simulink model "ieee80211n"  (Simulink 6.0)
settings: Solver=VariableStepDiscrete  StartTime=0.0  StopTime=inf  RelTol=1e-3
PreLoadFcn:
  | load IEEE80211n_init;
values from neighbouring files (symbols this model uses):
  params =     [IEEE80211n_init.mat]    (also in IEEE80211n_settings.m = p)
undefined symbols (not defined in the file or in its folder): magnitude
libraries: commblkintrlv2 x196, dspsigops x143, simulink x136, commdigbbndam2 x98, dspmtrx3 x96, dspsigattribs x69, dspstat3 x38, commutil2 x32, commsequence2 x26, commcnvcod2 x10, dspindex x9, dspmlti3 x8
(part 6 of 12)

== system ieee80211n/training sequence4/training sequence1 ==
  Frame Status Conversion1 : dspsigattribs/Frame Status Conversion  growRefPort=off  outframe=Frame-based
  Short Train sequence : Constant  Value=repmat(params.short_training_seq, [1 params.OFDM_LSTF_SymPerFrame])
  out : Outport
  wires:
  Short Train sequence/1 -> Frame Status Conversion1/1
  Frame Status Conversion1/1 -> out/1

== system ieee80211n/training sequence4/training sequence2 ==
  Frame Status Conversion{,1..3} (4 alike) : dspsigattribs/Frame Status Conversion  growRefPort=off  outframe=Frame-based
  "HT-LTF, 20MHz SS1" : Constant  Value=params.HT20_long_training_seq_ss1
  "HT-LTF, 20MHz SS2" : Constant  Value=params.HT20_long_training_seq_ss2
  "HT-LTF, 20MHz SS3" : Constant  Value=params.HT20_long_training_seq_ss3
  "HT-LTF, 20MHz SS4" : Constant  Value=params.HT20_long_training_seq_ss4
  "out, SS1" : Outport
  "out, SS2" : Outport  Port=2
  "out, SS3" : Outport  Port=3
  "out, SS4" : Outport  Port=4
  wires:
  "HT-LTF, 20MHz SS1"/1 -> Frame Status Conversion/1
  Frame Status Conversion/1 -> "out, SS1"/1
  "HT-LTF, 20MHz SS2"/1 -> Frame Status Conversion1/1
  Frame Status Conversion1/1 -> "out, SS2"/1
  "HT-LTF, 20MHz SS3"/1 -> Frame Status Conversion2/1
  Frame Status Conversion2/1 -> "out, SS3"/1
  "HT-LTF, 20MHz SS4"/1 -> Frame Status Conversion3/1
  Frame Status Conversion3/1 -> "out, SS4"/1

== system ieee80211n/training sequence4/training sequence3 ==
  Frame Status Conversion{,1..3} (4 alike) : dspsigattribs/Frame Status Conversion  growRefPort=off  outframe=Frame-based
  "HT-STF, 20MHz SS1" : Constant  Value=repmat(params.HT20_short_training_seq_ss1, [1 params.OFDM_HTSTF_SymPerFrame])
  "HT-STF, 20MHz SS2" : Constant  Value=repmat(params.HT20_short_training_seq_ss2, [1 params.OFDM_HTSTF_SymPerFrame])
  "HT-STF, 20MHz SS3" : Constant  Value=repmat(params.HT20_short_training_seq_ss3, [1 params.OFDM_HTSTF_SymPerFrame])
  "HT-STF, 20MHz SS4" : Constant  Value=repmat(params.HT20_short_training_seq_ss4, [1 params.OFDM_HTSTF_SymPerFrame])
  "out, SS1" : Outport
  "out, SS2" : Outport  Port=2
  "out, SS3" : Outport  Port=3
  "out, SS4" : Outport  Port=4
  wires:
  "HT-STF, 20MHz SS1"/1 -> Frame Status Conversion/1
  Frame Status Conversion/1 -> "out, SS1"/1
  "HT-STF, 20MHz SS2"/1 -> Frame Status Conversion1/1
  Frame Status Conversion1/1 -> "out, SS2"/1
  "HT-STF, 20MHz SS3"/1 -> Frame Status Conversion2/1
  Frame Status Conversion2/1 -> "out, SS3"/1
  "HT-STF, 20MHz SS4"/1 -> Frame Status Conversion3/1
  Frame Status Conversion3/1 -> "out, SS4"/1

== system ieee80211n/Demodbank/DecodeBankViterbi/Demodulator 1 ==
  rxsig : Inport  Port=1  LatchInput=off
  Enable : EnablePort
  Input bits : S-Function  AncestorBlock=dspindex/Multiport Selector  FunctionName=sdspmultiportsel  Parameters=rowsOrCols, numOutports, flatIdxVect, flatLenVect, idxErrMode  mask(Multiport Selector){rowsOrCols=Rows, idxCellArray={1:4*params.maxTxBitsPerBlock}, idxErrMode=Clip Index}
      mask prompts: rowsOrCols "Select:"; idxCellArray "Indices to output:"; idxErrMode "Invalid index:"
      mask help: Output specified rows or columns to one or more output ports. The number of output ports is determined by the number of index vectors, each specified as a separate vector entry in a cell array. Indices are 1-based and need not be unique.
      mask init:
      | [numOutports, flatLenVect, flatIdxVect] = dspblkmultiportsel(idxCellArray);
      mask Help: web(dspbhelp);
      mask StyleString: popup(Rows|Columns),edit,popup(Clip Index|Clip and Warn|Generate Error)
      mask Display: disp(['Select\n' &1]);
  Insert Zero1 : commsequence2/Insert Zero  insertZeroVector=punctureVector
  Insert Zero2 : commsequence2/Insert Zero  insertZeroVector=punctureVector
  Metric scaling : S-Function  AncestorBlock=dspindex/Multiport Selector  FunctionName=sdspmultiportsel  Parameters=rowsOrCols, numOutports, flatIdxVect, flatLenVect, idxErrMode  mask(Multiport Selector){rowsOrCols=Rows, idxCellArray={(1+4*params.maxTxBitsPerBlock):(2*4*params.maxTxBitsPerBlock)}, idxErrMode=Clip Index}
      mask prompts: rowsOrCols "Select:"; idxCellArray "Indices to output:"; idxErrMode "Invalid index:"
      mask help: Output specified rows or columns to one or more output ports. The number of output ports is determined by the number of index vectors, each specified as a separate vector entry in a cell array. Indices are 1-based and need not be unique.
      mask init:
      | [numOutports, flatLenVect, flatIdxVect] = dspblkmultiportsel(idxCellArray);
      mask Help: web(dspbhelp);
      mask StyleString: popup(Rows|Columns),edit,popup(Clip Index|Clip and Warn|Generate Error)
      mask Display: disp(['Select\n' &1]);
  Viterbi Decoder1 : S-Function  AncestorBlock=commcnvcod2/Viterbi Decoder  FunctionName=scomviterbi2  Parameters=S.k,S.n,S.numStates,S.outputs,S.nextStates, dectype, nsdecb, tbdepth, opmode, reset, mscale  mask(Viterbi Decoder){trellis=trellisStructure, dectype=Unquantized, nsdecb=4, tbdepth=vtbd, opmode=Continuous, reset=off, mscale=on}
      mask prompts: trellis "Trellis structure:"; dectype "Decision type:"; nsdecb "Number of soft decision bits:"; tbdepth "Traceback depth:"; opmode "Operation mode:"; reset "Reset input"; mscale "Use metric scaling input:"
      mask help: Uses the Viterbi algorithm to decode convolutionally encoded input data. Use the poly2trellis function to create a trellis using the constraint length, code generator (octal) and feedback connection (octal).
      mask init:
      | S= commblkviterbi(gcb,1,'init',trellis);
      | if ~isempty(S.status), error(S.status); end;
      | if opmode~=1, reset=0; end;
      mask Help: helpview(commbhelp)
      mask StyleString: edit,popup(Unquantized|Hard Decision|Soft Decision),edit,edit,popup(Continuous|Truncated|Terminated),checkbox,checkbox
      mask CallbackString: |commblkviterbi(gcb,1,'cbDecType');|||commblkviterbi(gcb,1,'cbOpMode');||
      mask Display:
      | plot(-5,-5,100,100,S.draw.x,S.draw.y);
      | disp('\nViterbi Decoder');
      | port_label('input',S.draw.p.i1,S.draw.p.i1s);
      | port_label('input',S.draw.p.i2,S.draw.p.i2s);
      | port_label('output',S.draw.p.o1,S.draw.p.o1s);
  Zero Pad2 : dspsigops/Zero Pad  padSigAt=End  zpadAlong=Columns  padNumOutRowsSpecMethod=User-specified  numOutRows=Nb  padNumOutColsSpecMethod=User-specified  numOutCols=1  trunc_flag=None
      settings: AttributesFormatString=\n
  Zero Pad3 : dspsigops/Zero Pad  padSigAt=End  zpadAlong=Columns  padNumOutRowsSpecMethod=User-specified  numOutRows=Nb  padNumOutColsSpecMethod=User-specified  numOutCols=1  trunc_flag=None
      settings: AttributesFormatString=\n
  rxdata : Outport  OutputWhenDisabled=reset  InitialOutput=0
  wires:
  Viterbi Decoder1/1 -> rxdata/1
  Zero Pad2/1 -> Insert Zero1/1
  Input bits/1 -> Zero Pad2/1
  Zero Pad3/1 -> Insert Zero2/1
  Metric scaling/1 -> Zero Pad3/1
  Insert Zero1/1 -> Viterbi Decoder1/1
  rxsig/1 -> Input bits/1, Metric scaling/1
  Insert Zero2/1 -> Viterbi Decoder1/2

== system ieee80211n/Demodbank/DecodeBankViterbi/Demodulator 2 ==
  rxsig : Inport  Port=1  LatchInput=off
  Enable : EnablePort
  Input bits : S-Function  AncestorBlock=dspindex/Multiport Selector  FunctionName=sdspmultiportsel  Parameters=rowsOrCols, numOutports, flatIdxVect, flatLenVect, idxErrMode  mask(Multiport Selector){rowsOrCols=Rows, idxCellArray={1:4*params.maxTxBitsPerBlock}, idxErrMode=Clip Index}
      mask prompts: rowsOrCols "Select:"; idxCellArray "Indices to output:"; idxErrMode "Invalid index:"
      mask help: Output specified rows or columns to one or more output ports. The number of output ports is determined by the number of index vectors, each specified as a separate vector entry in a cell array. Indices are 1-based and need not be unique.
      mask init:
      | [numOutports, flatLenVect, flatIdxVect] = dspblkmultiportsel(idxCellArray);
      mask Help: web(dspbhelp);
      mask StyleString: popup(Rows|Columns),edit,popup(Clip Index|Clip and Warn|Generate Error)
      mask Display: disp(['Select\n' &1]);
  Insert Zero1 : commsequence2/Insert Zero  insertZeroVector=punctureVector
  Insert Zero2 : commsequence2/Insert Zero  insertZeroVector=punctureVector
  Metric scaling : S-Function  AncestorBlock=dspindex/Multiport Selector  FunctionName=sdspmultiportsel  Parameters=rowsOrCols, numOutports, flatIdxVect, flatLenVect, idxErrMode  mask(Multiport Selector){rowsOrCols=Rows, idxCellArray={(1+4*params.maxTxBitsPerBlock):(2*4*params.maxTxBitsPerBlock)}, idxErrMode=Clip Index}
      mask prompts: rowsOrCols "Select:"; idxCellArray "Indices to output:"; idxErrMode "Invalid index:"
      mask help: Output specified rows or columns to one or more output ports. The number of output ports is determined by the number of index vectors, each specified as a separate vector entry in a cell array. Indices are 1-based and need not be unique.
      mask init:
      | [numOutports, flatLenVect, flatIdxVect] = dspblkmultiportsel(idxCellArray);
      mask Help: web(dspbhelp);
      mask StyleString: popup(Rows|Columns),edit,popup(Clip Index|Clip and Warn|Generate Error)
      mask Display: disp(['Select\n' &1]);
  Viterbi Decoder1 : S-Function  AncestorBlock=commcnvcod2/Viterbi Decoder  FunctionName=scomviterbi2  Parameters=S.k,S.n,S.numStates,S.outputs,S.nextStates, dectype, nsdecb, tbdepth, opmode, reset, mscale  mask(Viterbi Decoder){trellis=trellisStructure, dectype=Unquantized, nsdecb=4, tbdepth=vtbd, opmode=Continuous, reset=off, mscale=on}
      mask prompts: trellis "Trellis structure:"; dectype "Decision type:"; nsdecb "Number of soft decision bits:"; tbdepth "Traceback depth:"; opmode "Operation mode:"; reset "Reset input"; mscale "Use metric scaling input:"
      mask help: Uses the Viterbi algorithm to decode convolutionally encoded input data. Use the poly2trellis function to create a trellis using the constraint length, code generator (octal) and feedback connection (octal).
      mask init:
      | S= commblkviterbi(gcb,1,'init',trellis);
      | if ~isempty(S.status), error(S.status); end;
      | if opmode~=1, reset=0; end;
      mask Help: helpview(commbhelp)
      mask StyleString: edit,popup(Unquantized|Hard Decision|Soft Decision),edit,edit,popup(Continuous|Truncated|Terminated),checkbox,checkbox
      mask CallbackString: |commblkviterbi(gcb,1,'cbDecType');|||commblkviterbi(gcb,1,'cbOpMode');||
      mask Display:
      | plot(-5,-5,100,100,S.draw.x,S.draw.y);
      | disp('\nViterbi Decoder');
      | port_label('input',S.draw.p.i1,S.draw.p.i1s);
      | port_label('input',S.draw.p.i2,S.draw.p.i2s);
      | port_label('output',S.draw.p.o1,S.draw.p.o1s);
  Zero Pad2 : dspsigops/Zero Pad  padSigAt=End  zpadAlong=Columns  padNumOutRowsSpecMethod=User-specified  numOutRows=Nb  padNumOutColsSpecMethod=User-specified  numOutCols=1  trunc_flag=None
      settings: AttributesFormatString=\n
  Zero Pad3 : dspsigops/Zero Pad  padSigAt=End  zpadAlong=Columns  padNumOutRowsSpecMethod=User-specified  numOutRows=Nb  padNumOutColsSpecMethod=User-specified  numOutCols=1  trunc_flag=None
      settings: AttributesFormatString=\n
  rxdata : Outport  OutputWhenDisabled=reset  InitialOutput=0
  wires:
  Viterbi Decoder1/1 -> rxdata/1
  Zero Pad2/1 -> Insert Zero1/1
  Input bits/1 -> Zero Pad2/1
  Zero Pad3/1 -> Insert Zero2/1
  Metric scaling/1 -> Zero Pad3/1
  Insert Zero1/1 -> Viterbi Decoder1/1
  rxsig/1 -> Input bits/1, Metric scaling/1
  Insert Zero2/1 -> Viterbi Decoder1/2

== system ieee80211n/Demodbank/DecodeBankViterbi/Demodulator 3 ==
  rxsig : Inport  Port=1  LatchInput=off
  Enable : EnablePort
  Input bits : S-Function  AncestorBlock=dspindex/Multiport Selector  FunctionName=sdspmultiportsel  Parameters=rowsOrCols, numOutports, flatIdxVect, flatLenVect, idxErrMode  mask(Multiport Selector){rowsOrCols=Rows, idxCellArray={1:4*params.maxTxBitsPerBlock}, idxErrMode=Clip Index}
      mask prompts: rowsOrCols "Select:"; idxCellArray "Indices to output:"; idxErrMode "Invalid index:"
      mask help: Output specified rows or columns to one or more output ports. The number of output ports is determined by the number of index vectors, each specified as a separate vector entry in a cell array. Indices are 1-based and need not be unique.
      mask init:
      | [numOutports, flatLenVect, flatIdxVect] = dspblkmultiportsel(idxCellArray);
      mask Help: web(dspbhelp);
      mask StyleString: popup(Rows|Columns),edit,popup(Clip Index|Clip and Warn|Generate Error)
      mask Display: disp(['Select\n' &1]);
  Insert Zero1 : commsequence2/Insert Zero  insertZeroVector=punctureVector
  Insert Zero2 : commsequence2/Insert Zero  insertZeroVector=punctureVector
  Metric scaling : S-Function  AncestorBlock=dspindex/Multiport Selector  FunctionName=sdspmultiportsel  Parameters=rowsOrCols, numOutports, flatIdxVect, flatLenVect, idxErrMode  mask(Multiport Selector){rowsOrCols=Rows, idxCellArray={(1+4*params.maxTxBitsPerBlock):(2*4*params.maxTxBitsPerBlock)}, idxErrMode=Clip Index}
      mask prompts: rowsOrCols "Select:"; idxCellArray "Indices to output:"; idxErrMode "Invalid index:"
      mask help: Output specified rows or columns to one or more output ports. The number of output ports is determined by the number of index vectors, each specified as a separate vector entry in a cell array. Indices are 1-based and need not be unique.
      mask init:
      | [numOutports, flatLenVect, flatIdxVect] = dspblkmultiportsel(idxCellArray);
      mask Help: web(dspbhelp);
      mask StyleString: popup(Rows|Columns),edit,popup(Clip Index|Clip and Warn|Generate Error)
      mask Display: disp(['Select\n' &1]);
  Viterbi Decoder1 : S-Function  AncestorBlock=commcnvcod2/Viterbi Decoder  FunctionName=scomviterbi2  Parameters=S.k,S.n,S.numStates,S.outputs,S.nextStates, dectype, nsdecb, tbdepth, opmode, reset, mscale  mask(Viterbi Decoder){trellis=trellisStructure, dectype=Unquantized, nsdecb=4, tbdepth=vtbd, opmode=Continuous, reset=off, mscale=on}
      mask prompts: trellis "Trellis structure:"; dectype "Decision type:"; nsdecb "Number of soft decision bits:"; tbdepth "Traceback depth:"; opmode "Operation mode:"; reset "Reset input"; mscale "Use metric scaling input:"
      mask help: Uses the Viterbi algorithm to decode convolutionally encoded input data. Use the poly2trellis function to create a trellis using the constraint length, code generator (octal) and feedback connection (octal).
      mask init:
      | S= commblkviterbi(gcb,1,'init',trellis);
      | if ~isempty(S.status), error(S.status); end;
      | if opmode~=1, reset=0; end;
      mask Help: helpview(commbhelp)
      mask StyleString: edit,popup(Unquantized|Hard Decision|Soft Decision),edit,edit,popup(Continuous|Truncated|Terminated),checkbox,checkbox
      mask CallbackString: |commblkviterbi(gcb,1,'cbDecType');|||commblkviterbi(gcb,1,'cbOpMode');||
      mask Display:
      | plot(-5,-5,100,100,S.draw.x,S.draw.y);
      | disp('\nViterbi Decoder');
      | port_label('input',S.draw.p.i1,S.draw.p.i1s);
      | port_label('input',S.draw.p.i2,S.draw.p.i2s);
      | port_label('output',S.draw.p.o1,S.draw.p.o1s);
  Zero Pad2 : dspsigops/Zero Pad  padSigAt=End  zpadAlong=Columns  padNumOutRowsSpecMethod=User-specified  numOutRows=Nb  padNumOutColsSpecMethod=User-specified  numOutCols=1  trunc_flag=None
      settings: AttributesFormatString=\n
  Zero Pad3 : dspsigops/Zero Pad  padSigAt=End  zpadAlong=Columns  padNumOutRowsSpecMethod=User-specified  numOutRows=Nb  padNumOutColsSpecMethod=User-specified  numOutCols=1  trunc_flag=None
      settings: AttributesFormatString=\n
  rxdata : Outport  OutputWhenDisabled=reset  InitialOutput=0
  wires:
  Viterbi Decoder1/1 -> rxdata/1
  Zero Pad2/1 -> Insert Zero1/1
  Input bits/1 -> Zero Pad2/1
  Zero Pad3/1 -> Insert Zero2/1
  Metric scaling/1 -> Zero Pad3/1
  Insert Zero1/1 -> Viterbi Decoder1/1
  rxsig/1 -> Input bits/1, Metric scaling/1
  Insert Zero2/1 -> Viterbi Decoder1/2

== system ieee80211n/Demodbank/DecodeBankViterbi/Demodulator 4 ==
  rxsig : Inport  Port=1  LatchInput=off
  Enable : EnablePort
  Input bits : S-Function  AncestorBlock=dspindex/Multiport Selector  FunctionName=sdspmultiportsel  Parameters=rowsOrCols, numOutports, flatIdxVect, flatLenVect, idxErrMode  mask(Multiport Selector){rowsOrCols=Rows, idxCellArray={1:4*params.maxTxBitsPerBlock}, idxErrMode=Clip Index}
      mask prompts: rowsOrCols "Select:"; idxCellArray "Indices to output:"; idxErrMode "Invalid index:"
      mask help: Output specified rows or columns to one or more output ports. The number of output ports is determined by the number of index vectors, each specified as a separate vector entry in a cell array. Indices are 1-based and need not be unique.
      mask init:
      | [numOutports, flatLenVect, flatIdxVect] = dspblkmultiportsel(idxCellArray);
      mask Help: web(dspbhelp);
      mask StyleString: popup(Rows|Columns),edit,popup(Clip Index|Clip and Warn|Generate Error)
      mask Display: disp(['Select\n' &1]);
  Insert Zero1 : commsequence2/Insert Zero  insertZeroVector=punctureVector
  Insert Zero2 : commsequence2/Insert Zero  insertZeroVector=punctureVector
  Metric scaling : S-Function  AncestorBlock=dspindex/Multiport Selector  FunctionName=sdspmultiportsel  Parameters=rowsOrCols, numOutports, flatIdxVect, flatLenVect, idxErrMode  mask(Multiport Selector){rowsOrCols=Rows, idxCellArray={(1+4*params.maxTxBitsPerBlock):(2*4*params.maxTxBitsPerBlock)}, idxErrMode=Clip Index}
      mask prompts: rowsOrCols "Select:"; idxCellArray "Indices to output:"; idxErrMode "Invalid index:"
      mask help: Output specified rows or columns to one or more output ports. The number of output ports is determined by the number of index vectors, each specified as a separate vector entry in a cell array. Indices are 1-based and need not be unique.
      mask init:
      | [numOutports, flatLenVect, flatIdxVect] = dspblkmultiportsel(idxCellArray);
      mask Help: web(dspbhelp);
      mask StyleString: popup(Rows|Columns),edit,popup(Clip Index|Clip and Warn|Generate Error)
      mask Display: disp(['Select\n' &1]);
  Viterbi Decoder1 : S-Function  AncestorBlock=commcnvcod2/Viterbi Decoder  FunctionName=scomviterbi2  Parameters=S.k,S.n,S.numStates,S.outputs,S.nextStates, dectype, nsdecb, tbdepth, opmode, reset, mscale  mask(Viterbi Decoder){trellis=trellisStructure, dectype=Unquantized, nsdecb=4, tbdepth=vtbd, opmode=Continuous, reset=off, mscale=on}
      mask prompts: trellis "Trellis structure:"; dectype "Decision type:"; nsdecb "Number of soft decision bits:"; tbdepth "Traceback depth:"; opmode "Operation mode:"; reset "Reset input"; mscale "Use metric scaling input:"
      mask help: Uses the Viterbi algorithm to decode convolutionally encoded input data. Use the poly2trellis function to create a trellis using the constraint length, code generator (octal) and feedback connection (octal).
      mask init:
      | S= commblkviterbi(gcb,1,'init',trellis);
      | if ~isempty(S.status), error(S.status); end;
      | if opmode~=1, reset=0; end;
      mask Help: helpview(commbhelp)
      mask StyleString: edit,popup(Unquantized|Hard Decision|Soft Decision),edit,edit,popup(Continuous|Truncated|Terminated),checkbox,checkbox
      mask CallbackString: |commblkviterbi(gcb,1,'cbDecType');|||commblkviterbi(gcb,1,'cbOpMode');||
      mask Display:
      | plot(-5,-5,100,100,S.draw.x,S.draw.y);
      | disp('\nViterbi Decoder');
      | port_label('input',S.draw.p.i1,S.draw.p.i1s);
      | port_label('input',S.draw.p.i2,S.draw.p.i2s);
      | port_label('output',S.draw.p.o1,S.draw.p.o1s);
  Zero Pad2 : dspsigops/Zero Pad  padSigAt=End  zpadAlong=Columns  padNumOutRowsSpecMethod=User-specified  numOutRows=Nb  padNumOutColsSpecMethod=User-specified  numOutCols=1  trunc_flag=None
      settings: AttributesFormatString=\n
  Zero Pad3 : dspsigops/Zero Pad  padSigAt=End  zpadAlong=Columns  padNumOutRowsSpecMethod=User-specified  numOutRows=Nb  padNumOutColsSpecMethod=User-specified  numOutCols=1  trunc_flag=None
      settings: AttributesFormatString=\n
  rxdata : Outport  OutputWhenDisabled=reset  InitialOutput=0
  wires:
  Viterbi Decoder1/1 -> rxdata/1
  rxsig/1 -> Input bits/1, Metric scaling/1
  Zero Pad2/1 -> Insert Zero1/1
  Input bits/1 -> Zero Pad2/1
  Zero Pad3/1 -> Insert Zero2/1
  Metric scaling/1 -> Zero Pad3/1
  Insert Zero1/1 -> Viterbi Decoder1/1
  Insert Zero2/1 -> Viterbi Decoder1/2

== system ieee80211n/Demodbank/DecodeBankViterbi/Demodulator 5 ==
  rxsig : Inport  Port=1  LatchInput=off
  Enable : EnablePort
  Input bits : S-Function  AncestorBlock=dspindex/Multiport Selector  FunctionName=sdspmultiportsel  Parameters=rowsOrCols, numOutports, flatIdxVect, flatLenVect, idxErrMode  mask(Multiport Selector){rowsOrCols=Rows, idxCellArray={1:4*params.maxTxBitsPerBlock}, idxErrMode=Clip Index}
      mask prompts: rowsOrCols "Select:"; idxCellArray "Indices to output:"; idxErrMode "Invalid index:"
      mask help: Output specified rows or columns to one or more output ports. The number of output ports is determined by the number of index vectors, each specified as a separate vector entry in a cell array. Indices are 1-based and need not be unique.
      mask init:
      | [numOutports, flatLenVect, flatIdxVect] = dspblkmultiportsel(idxCellArray);
      mask Help: web(dspbhelp);
      mask StyleString: popup(Rows|Columns),edit,popup(Clip Index|Clip and Warn|Generate Error)
      mask Display: disp(['Select\n' &1]);
  Insert Zero1 : commsequence2/Insert Zero  insertZeroVector=punctureVector
  Insert Zero2 : commsequence2/Insert Zero  insertZeroVector=punctureVector
  Metric scaling : S-Function  AncestorBlock=dspindex/Multiport Selector  FunctionName=sdspmultiportsel  Parameters=rowsOrCols, numOutports, flatIdxVect, flatLenVect, idxErrMode  mask(Multiport Selector){rowsOrCols=Rows, idxCellArray={(1+4*params.maxTxBitsPerBlock):(2*4*params.maxTxBitsPerBlock)}, idxErrMode=Clip Index}
      mask prompts: rowsOrCols "Select:"; idxCellArray "Indices to output:"; idxErrMode "Invalid index:"
      mask help: Output specified rows or columns to one or more output ports. The number of output ports is determined by the number of index vectors, each specified as a separate vector entry in a cell array. Indices are 1-based and need not be unique.
      mask init:
      | [numOutports, flatLenVect, flatIdxVect] = dspblkmultiportsel(idxCellArray);
      mask Help: web(dspbhelp);
      mask StyleString: popup(Rows|Columns),edit,popup(Clip Index|Clip and Warn|Generate Error)
      mask Display: disp(['Select\n' &1]);
  Viterbi Decoder1 : S-Function  AncestorBlock=commcnvcod2/Viterbi Decoder  FunctionName=scomviterbi2  Parameters=S.k,S.n,S.numStates,S.outputs,S.nextStates, dectype, nsdecb, tbdepth, opmode, reset, mscale  mask(Viterbi Decoder){trellis=trellisStructure, dectype=Unquantized, nsdecb=4, tbdepth=vtbd, opmode=Continuous, reset=off, mscale=on}
      mask prompts: trellis "Trellis structure:"; dectype "Decision type:"; nsdecb "Number of soft decision bits:"; tbdepth "Traceback depth:"; opmode "Operation mode:"; reset "Reset input"; mscale "Use metric scaling input:"
      mask help: Uses the Viterbi algorithm to decode convolutionally encoded input data. Use the poly2trellis function to create a trellis using the constraint length, code generator (octal) and feedback connection (octal).
      mask init:
      | S= commblkviterbi(gcb,1,'init',trellis);
      | if ~isempty(S.status), error(S.status); end;
      | if opmode~=1, reset=0; end;
      mask Help: helpview(commbhelp)
      mask StyleString: edit,popup(Unquantized|Hard Decision|Soft Decision),edit,edit,popup(Continuous|Truncated|Terminated),checkbox,checkbox
      mask CallbackString: |commblkviterbi(gcb,1,'cbDecType');|||commblkviterbi(gcb,1,'cbOpMode');||
      mask Display:
      | plot(-5,-5,100,100,S.draw.x,S.draw.y);
      | disp('\nViterbi Decoder');
      | port_label('input',S.draw.p.i1,S.draw.p.i1s);
      | port_label('input',S.draw.p.i2,S.draw.p.i2s);
      | port_label('output',S.draw.p.o1,S.draw.p.o1s);
  Zero Pad2 : dspsigops/Zero Pad  padSigAt=End  zpadAlong=Columns  padNumOutRowsSpecMethod=User-specified  numOutRows=Nb  padNumOutColsSpecMethod=User-specified  numOutCols=1  trunc_flag=None
      settings: AttributesFormatString=\n
  Zero Pad3 : dspsigops/Zero Pad  padSigAt=End  zpadAlong=Columns  padNumOutRowsSpecMethod=User-specified  numOutRows=Nb  padNumOutColsSpecMethod=User-specified  numOutCols=1  trunc_flag=None
      settings: AttributesFormatString=\n
  rxdata : Outport  OutputWhenDisabled=reset  InitialOutput=0
  wires:
  Viterbi Decoder1/1 -> rxdata/1
  rxsig/1 -> Input bits/1, Metric scaling/1
  Zero Pad2/1 -> Insert Zero1/1
  Input bits/1 -> Zero Pad2/1
  Zero Pad3/1 -> Insert Zero2/1
  Metric scaling/1 -> Zero Pad3/1
  Insert Zero1/1 -> Viterbi Decoder1/1
  Insert Zero2/1 -> Viterbi Decoder1/2

== system ieee80211n/Demodbank/DecodeBankViterbi/Demodulator 6 ==
  rxsig : Inport  Port=1  LatchInput=off
  Enable : EnablePort
  Input bits : S-Function  AncestorBlock=dspindex/Multiport Selector  FunctionName=sdspmultiportsel  Parameters=rowsOrCols, numOutports, flatIdxVect, flatLenVect, idxErrMode  mask(Multiport Selector){rowsOrCols=Rows, idxCellArray={1:4*params.maxTxBitsPerBlock}, idxErrMode=Clip Index}
      mask prompts: rowsOrCols "Select:"; idxCellArray "Indices to output:"; idxErrMode "Invalid index:"
      mask help: Output specified rows or columns to one or more output ports. The number of output ports is determined by the number of index vectors, each specified as a separate vector entry in a cell array. Indices are 1-based and need not be unique.
      mask init:
      | [numOutports, flatLenVect, flatIdxVect] = dspblkmultiportsel(idxCellArray);
      mask Help: web(dspbhelp);
      mask StyleString: popup(Rows|Columns),edit,popup(Clip Index|Clip and Warn|Generate Error)
      mask Display: disp(['Select\n' &1]);
  Insert Zero1 : commsequence2/Insert Zero  insertZeroVector=punctureVector
  Insert Zero2 : commsequence2/Insert Zero  insertZeroVector=punctureVector
  Metric scaling : S-Function  AncestorBlock=dspindex/Multiport Selector  FunctionName=sdspmultiportsel  Parameters=rowsOrCols, numOutports, flatIdxVect, flatLenVect, idxErrMode  mask(Multiport Selector){rowsOrCols=Rows, idxCellArray={(1+4*params.maxTxBitsPerBlock):(2*4*params.maxTxBitsPerBlock)}, idxErrMode=Clip Index}
      mask prompts: rowsOrCols "Select:"; idxCellArray "Indices to output:"; idxErrMode "Invalid index:"
      mask help: Output specified rows or columns to one or more output ports. The number of output ports is determined by the number of index vectors, each specified as a separate vector entry in a cell array. Indices are 1-based and need not be unique.
      mask init:
      | [numOutports, flatLenVect, flatIdxVect] = dspblkmultiportsel(idxCellArray);
      mask Help: web(dspbhelp);
      mask StyleString: popup(Rows|Columns),edit,popup(Clip Index|Clip and Warn|Generate Error)
      mask Display: disp(['Select\n' &1]);
  Viterbi Decoder1 : S-Function  AncestorBlock=commcnvcod2/Viterbi Decoder  FunctionName=scomviterbi2  Parameters=S.k,S.n,S.numStates,S.outputs,S.nextStates, dectype, nsdecb, tbdepth, opmode, reset, mscale  mask(Viterbi Decoder){trellis=trellisStructure, dectype=Unquantized, nsdecb=4, tbdepth=vtbd, opmode=Continuous, reset=off, mscale=on}
      mask prompts: trellis "Trellis structure:"; dectype "Decision type:"; nsdecb "Number of soft decision bits:"; tbdepth "Traceback depth:"; opmode "Operation mode:"; reset "Reset input"; mscale "Use metric scaling input:"
      mask help: Uses the Viterbi algorithm to decode convolutionally encoded input data. Use the poly2trellis function to create a trellis using the constraint length, code generator (octal) and feedback connection (octal).
      mask init:
      | S= commblkviterbi(gcb,1,'init',trellis);
      | if ~isempty(S.status), error(S.status); end;
      | if opmode~=1, reset=0; end;
      mask Help: helpview(commbhelp)
      mask StyleString: edit,popup(Unquantized|Hard Decision|Soft Decision),edit,edit,popup(Continuous|Truncated|Terminated),checkbox,checkbox
      mask CallbackString: |commblkviterbi(gcb,1,'cbDecType');|||commblkviterbi(gcb,1,'cbOpMode');||
      mask Display:
      | plot(-5,-5,100,100,S.draw.x,S.draw.y);
      | disp('\nViterbi Decoder');
      | port_label('input',S.draw.p.i1,S.draw.p.i1s);
      | port_label('input',S.draw.p.i2,S.draw.p.i2s);
      | port_label('output',S.draw.p.o1,S.draw.p.o1s);
  Zero Pad2 : dspsigops/Zero Pad  padSigAt=End  zpadAlong=Columns  padNumOutRowsSpecMethod=User-specified  numOutRows=Nb  padNumOutColsSpecMethod=User-specified  numOutCols=1  trunc_flag=None
      settings: AttributesFormatString=\n
  Zero Pad3 : dspsigops/Zero Pad  padSigAt=End  zpadAlong=Columns  padNumOutRowsSpecMethod=User-specified  numOutRows=Nb  padNumOutColsSpecMethod=User-specified  numOutCols=1  trunc_flag=None
      settings: AttributesFormatString=\n
  rxdata : Outport  OutputWhenDisabled=reset  InitialOutput=0
  wires:
  Viterbi Decoder1/1 -> rxdata/1
  Zero Pad2/1 -> Insert Zero1/1
  Input bits/1 -> Zero Pad2/1
  Zero Pad3/1 -> Insert Zero2/1
  Metric scaling/1 -> Zero Pad3/1
  Insert Zero1/1 -> Viterbi Decoder1/1
  rxsig/1 -> Input bits/1, Metric scaling/1
  Insert Zero2/1 -> Viterbi Decoder1/2

== system ieee80211n/Demodbank/DecodeBankViterbi/Demodulator 7 ==
  rxsig : Inport  Port=1  LatchInput=off
  Enable : EnablePort
  Input bits : S-Function  AncestorBlock=dspindex/Multiport Selector  FunctionName=sdspmultiportsel  Parameters=rowsOrCols, numOutports, flatIdxVect, flatLenVect, idxErrMode  mask(Multiport Selector){rowsOrCols=Rows, idxCellArray={1:4*params.maxTxBitsPerBlock}, idxErrMode=Clip Index}
      mask prompts: rowsOrCols "Select:"; idxCellArray "Indices to output:"; idxErrMode "Invalid index:"
      mask help: Output specified rows or columns to one or more output ports. The number of output ports is determined by the number of index vectors, each specified as a separate vector entry in a cell array. Indices are 1-based and need not be unique.
      mask init:
      | [numOutports, flatLenVect, flatIdxVect] = dspblkmultiportsel(idxCellArray);
      mask Help: web(dspbhelp);
      mask StyleString: popup(Rows|Columns),edit,popup(Clip Index|Clip and Warn|Generate Error)
      mask Display: disp(['Select\n' &1]);
  Insert Zero1 : commsequence2/Insert Zero  insertZeroVector=punctureVector
  Insert Zero2 : commsequence2/Insert Zero  insertZeroVector=punctureVector
  Metric scaling : S-Function  AncestorBlock=dspindex/Multiport Selector  FunctionName=sdspmultiportsel  Parameters=rowsOrCols, numOutports, flatIdxVect, flatLenVect, idxErrMode  mask(Multiport Selector){rowsOrCols=Rows, idxCellArray={(1+4*params.maxTxBitsPerBlock):(2*4*params.maxTxBitsPerBlock)}, idxErrMode=Clip Index}
      mask prompts: rowsOrCols "Select:"; idxCellArray "Indices to output:"; idxErrMode "Invalid index:"
      mask help: Output specified rows or columns to one or more output ports. The number of output ports is determined by the number of index vectors, each specified as a separate vector entry in a cell array. Indices are 1-based and need not be unique.
      mask init:
      | [numOutports, flatLenVect, flatIdxVect] = dspblkmultiportsel(idxCellArray);
      mask Help: web(dspbhelp);
      mask StyleString: popup(Rows|Columns),edit,popup(Clip Index|Clip and Warn|Generate Error)
      mask Display: disp(['Select\n' &1]);
  Viterbi Decoder1 : S-Function  AncestorBlock=commcnvcod2/Viterbi Decoder  FunctionName=scomviterbi2  Parameters=S.k,S.n,S.numStates,S.outputs,S.nextStates, dectype, nsdecb, tbdepth, opmode, reset, mscale  mask(Viterbi Decoder){trellis=trellisStructure, dectype=Unquantized, nsdecb=4, tbdepth=vtbd, opmode=Continuous, reset=off, mscale=on}
      mask prompts: trellis "Trellis structure:"; dectype "Decision type:"; nsdecb "Number of soft decision bits:"; tbdepth "Traceback depth:"; opmode "Operation mode:"; reset "Reset input"; mscale "Use metric scaling input:"
      mask help: Uses the Viterbi algorithm to decode convolutionally encoded input data. Use the poly2trellis function to create a trellis using the constraint length, code generator (octal) and feedback connection (octal).
      mask init:
      | S= commblkviterbi(gcb,1,'init',trellis);
      | if ~isempty(S.status), error(S.status); end;
      | if opmode~=1, reset=0; end;
      mask Help: helpview(commbhelp)
      mask StyleString: edit,popup(Unquantized|Hard Decision|Soft Decision),edit,edit,popup(Continuous|Truncated|Terminated),checkbox,checkbox
      mask CallbackString: |commblkviterbi(gcb,1,'cbDecType');|||commblkviterbi(gcb,1,'cbOpMode');||
      mask Display:
      | plot(-5,-5,100,100,S.draw.x,S.draw.y);
      | disp('\nViterbi Decoder');
      | port_label('input',S.draw.p.i1,S.draw.p.i1s);
      | port_label('input',S.draw.p.i2,S.draw.p.i2s);
      | port_label('output',S.draw.p.o1,S.draw.p.o1s);
  Zero Pad2 : dspsigops/Zero Pad  padSigAt=End  zpadAlong=Columns  padNumOutRowsSpecMethod=User-specified  numOutRows=Nb  padNumOutColsSpecMethod=User-specified  numOutCols=1  trunc_flag=None
      settings: AttributesFormatString=\n
  Zero Pad3 : dspsigops/Zero Pad  padSigAt=End  zpadAlong=Columns  padNumOutRowsSpecMethod=User-specified  numOutRows=Nb  padNumOutColsSpecMethod=User-specified  numOutCols=1  trunc_flag=None
      settings: AttributesFormatString=\n
  rxdata : Outport  OutputWhenDisabled=reset  InitialOutput=0
  wires:
  Viterbi Decoder1/1 -> rxdata/1
  Zero Pad2/1 -> Insert Zero1/1
  Input bits/1 -> Zero Pad2/1
  Zero Pad3/1 -> Insert Zero2/1
  Metric scaling/1 -> Zero Pad3/1
  Insert Zero1/1 -> Viterbi Decoder1/1
  rxsig/1 -> Input bits/1, Metric scaling/1
  Insert Zero2/1 -> Viterbi Decoder1/2

== system ieee80211n/Demodbank/DecodeBankViterbi/Demodulator 8 ==
  rxsig : Inport  Port=1  LatchInput=off
  Enable : EnablePort
  Input bits : S-Function  AncestorBlock=dspindex/Multiport Selector  FunctionName=sdspmultiportsel  Parameters=rowsOrCols, numOutports, flatIdxVect, flatLenVect, idxErrMode  mask(Multiport Selector){rowsOrCols=Rows, idxCellArray={1:4*params.maxTxBitsPerBlock}, idxErrMode=Clip Index}
      mask prompts: rowsOrCols "Select:"; idxCellArray "Indices to output:"; idxErrMode "Invalid index:"
      mask help: Output specified rows or columns to one or more output ports. The number of output ports is determined by the number of index vectors, each specified as a separate vector entry in a cell array. Indices are 1-based and need not be unique.
      mask init:
      | [numOutports, flatLenVect, flatIdxVect] = dspblkmultiportsel(idxCellArray);
      mask Help: web(dspbhelp);
      mask StyleString: popup(Rows|Columns),edit,popup(Clip Index|Clip and Warn|Generate Error)
      mask Display: disp(['Select\n' &1]);
  Insert Zero1 : commsequence2/Insert Zero  insertZeroVector=punctureVector
  Insert Zero2 : commsequence2/Insert Zero  insertZeroVector=punctureVector
  Metric scaling : S-Function  AncestorBlock=dspindex/Multiport Selector  FunctionName=sdspmultiportsel  Parameters=rowsOrCols, numOutports, flatIdxVect, flatLenVect, idxErrMode  mask(Multiport Selector){rowsOrCols=Rows, idxCellArray={(1+4*params.maxTxBitsPerBlock):(2*4*params.maxTxBitsPerBlock)}, idxErrMode=Clip Index}
      mask prompts: rowsOrCols "Select:"; idxCellArray "Indices to output:"; idxErrMode "Invalid index:"
      mask help: Output specified rows or columns to one or more output ports. The number of output ports is determined by the number of index vectors, each specified as a separate vector entry in a cell array. Indices are 1-based and need not be unique.
      mask init:
      | [numOutports, flatLenVect, flatIdxVect] = dspblkmultiportsel(idxCellArray);
      mask Help: web(dspbhelp);
      mask StyleString: popup(Rows|Columns),edit,popup(Clip Index|Clip and Warn|Generate Error)
      mask Display: disp(['Select\n' &1]);
  Viterbi Decoder1 : S-Function  AncestorBlock=commcnvcod2/Viterbi Decoder  FunctionName=scomviterbi2  Parameters=S.k,S.n,S.numStates,S.outputs,S.nextStates, dectype, nsdecb, tbdepth, opmode, reset, mscale  mask(Viterbi Decoder){trellis=trellisStructure, dectype=Unquantized, nsdecb=4, tbdepth=vtbd, opmode=Continuous, reset=off, mscale=on}
      mask prompts: trellis "Trellis structure:"; dectype "Decision type:"; nsdecb "Number of soft decision bits:"; tbdepth "Traceback depth:"; opmode "Operation mode:"; reset "Reset input"; mscale "Use metric scaling input:"
      mask help: Uses the Viterbi algorithm to decode convolutionally encoded input data. Use the poly2trellis function to create a trellis using the constraint length, code generator (octal) and feedback connection (octal).
      mask init:
      | S= commblkviterbi(gcb,1,'init',trellis);
      | if ~isempty(S.status), error(S.status); end;
      | if opmode~=1, reset=0; end;
      mask Help: helpview(commbhelp)
      mask StyleString: edit,popup(Unquantized|Hard Decision|Soft Decision),edit,edit,popup(Continuous|Truncated|Terminated),checkbox,checkbox
      mask CallbackString: |commblkviterbi(gcb,1,'cbDecType');|||commblkviterbi(gcb,1,'cbOpMode');||
      mask Display:
      | plot(-5,-5,100,100,S.draw.x,S.draw.y);
      | disp('\nViterbi Decoder');
      | port_label('input',S.draw.p.i1,S.draw.p.i1s);
      | port_label('input',S.draw.p.i2,S.draw.p.i2s);
      | port_label('output',S.draw.p.o1,S.draw.p.o1s);
  Zero Pad2 : dspsigops/Zero Pad  padSigAt=End  zpadAlong=Columns  padNumOutRowsSpecMethod=User-specified  numOutRows=Nb  padNumOutColsSpecMethod=User-specified  numOutCols=1  trunc_flag=None
      settings: AttributesFormatString=\n
  Zero Pad3 : dspsigops/Zero Pad  padSigAt=End  zpadAlong=Columns  padNumOutRowsSpecMethod=User-specified  numOutRows=Nb  padNumOutColsSpecMethod=User-specified  numOutCols=1  trunc_flag=None
      settings: AttributesFormatString=\n
  rxdata : Outport  OutputWhenDisabled=reset  InitialOutput=0
  wires:
  Viterbi Decoder1/1 -> rxdata/1
  Zero Pad2/1 -> Insert Zero1/1
  Input bits/1 -> Zero Pad2/1
  Zero Pad3/1 -> Insert Zero2/1
  Metric scaling/1 -> Zero Pad3/1
  Insert Zero1/1 -> Viterbi Decoder1/1
  rxsig/1 -> Input bits/1, Metric scaling/1
  Insert Zero2/1 -> Viterbi Decoder1/2

== system ieee80211n/Demodbank/Demod_ss1/Demodulator 1 ==
  rxsig : Inport  Port=1  LatchInput=off
  mscale : Inport  Port=2  LatchInput=off
  Enable : EnablePort
  Bits Per Symbol : Constant  Value=ones(1, log2(modOrder))  VectorParams1D=off
  General Block Deinterleaver : commblkintrlv2/General Block Deinterleaver  elements=interleaverElements
  General Block Deinterleaver1 : commblkintrlv2/General Block Deinterleaver  elements=interleaverElements
  Matrix Deinterleaver : commblkintrlv2/Matrix Deinterleaver  Nrows=interleaverRows  Ncols=interleaverCols
  Matrix Deinterleaver1 : commblkintrlv2/Matrix Deinterleaver  Nrows=interleaverRows  Ncols=interleaverCols
  Matrix Multiply : Product  Multiplication=Matrix(*)
  Rectangular QAM Demodulator Baseband : commdigbbndam2/Rectangular QAM Demodulator Baseband  M=modOrder  OutType=Bit  Dec=Gray  PowType=Average Power  MinDist=2  AvgPow=1  PeakPow=1  Ph=0  numSamp=1
  Rectangular QAM Modulator Baseband1 : commdigbbndam2/Rectangular QAM Modulator Baseband  M=modOrder  InType=Bit  Enc=Gray  PowType=Average Power  MinDist=2  AvgPow=1  PeakPow=1  Ph=0  numSamp=1
  Reshape6 : simulink/Math Operations/Reshape  OutputDimensionality=Column vector  OutputDimensions=1600
  Sum : Sum  Inputs=|+-  SaturateOnIntegerOverflow=on
  Transpose : dspmtrx3/Transpose  Hermitian=off  overflowFlag=on
  Unipolar to Bipolar Converter2 : commutil2/Unipolar to Bipolar Converter  M=2  polarity=Negative
  rxdata : Outport  OutputWhenDisabled=reset  InitialOutput=0
  symerr : Outport  Port=2  OutputWhenDisabled=reset  InitialOutput=0
  mscale out : Outport  Port=3  OutputWhenDisabled=reset  InitialOutput=0
  wires:
  General Block Deinterleaver/1 -> Matrix Deinterleaver/1
  Matrix Deinterleaver/1 -> rxdata/1
  Sum/1 -> symerr/1
  Rectangular QAM Modulator Baseband1/1 -> Sum/1
  Unipolar to Bipolar Converter2/1 -> General Block Deinterleaver/1
  rxsig/1 -> Sum/2, Rectangular QAM Demodulator Baseband/1
  Rectangular QAM Demodulator Baseband/1 -> Rectangular QAM Modulator Baseband1/1, Unipolar to Bipolar Converter2/1
  General Block Deinterleaver1/1 -> Matrix Deinterleaver1/1
  Matrix Deinterleaver1/1 -> mscale out/1
  mscale/1 -> Matrix Multiply/1
  Matrix Multiply/1 -> Transpose/1
  Bits Per Symbol/1 -> Matrix Multiply/2
  Reshape6/1 -> General Block Deinterleaver1/1
  Transpose/1 -> Reshape6/1

== system ieee80211n/Demodbank/Demod_ss1/Demodulator 2 ==
  rxsig : Inport  Port=1  LatchInput=off
  mscale : Inport  Port=2  LatchInput=off
  Enable : EnablePort
  Bits Per Symbol : Constant  Value=ones(1, log2(modOrder))  VectorParams1D=off
  General Block Deinterleaver : commblkintrlv2/General Block Deinterleaver  elements=interleaverElements
  General Block Deinterleaver1 : commblkintrlv2/General Block Deinterleaver  elements=interleaverElements
  Matrix Deinterleaver : commblkintrlv2/Matrix Deinterleaver  Nrows=interleaverRows  Ncols=interleaverCols
  Matrix Deinterleaver1 : commblkintrlv2/Matrix Deinterleaver  Nrows=interleaverRows  Ncols=interleaverCols
  Matrix Multiply : Product  Multiplication=Matrix(*)
  Rectangular QAM Demodulator Baseband : commdigbbndam2/Rectangular QAM Demodulator Baseband  M=modOrder  OutType=Bit  Dec=Gray  PowType=Average Power  MinDist=2  AvgPow=1  PeakPow=1  Ph=0  numSamp=1
  Rectangular QAM Modulator Baseband1 : commdigbbndam2/Rectangular QAM Modulator Baseband  M=modOrder  InType=Bit  Enc=Gray  PowType=Average Power  MinDist=2  AvgPow=1  PeakPow=1  Ph=0  numSamp=1
  Reshape6 : simulink/Math Operations/Reshape  OutputDimensionality=Column vector  OutputDimensions=1600
  Sum : Sum  Inputs=|+-  SaturateOnIntegerOverflow=on
  Transpose : dspmtrx3/Transpose  Hermitian=off  overflowFlag=on
  Unipolar to Bipolar Converter2 : commutil2/Unipolar to Bipolar Converter  M=2  polarity=Negative
  rxdata : Outport  OutputWhenDisabled=reset  InitialOutput=0
  symerr : Outport  Port=2  OutputWhenDisabled=reset  InitialOutput=0
  mscale out : Outport  Port=3  OutputWhenDisabled=reset  InitialOutput=0
  wires:
  General Block Deinterleaver/1 -> Matrix Deinterleaver/1
  Matrix Deinterleaver/1 -> rxdata/1
  Sum/1 -> symerr/1
  Rectangular QAM Modulator Baseband1/1 -> Sum/1
  Unipolar to Bipolar Converter2/1 -> General Block Deinterleaver/1
  rxsig/1 -> Sum/2, Rectangular QAM Demodulator Baseband/1
  Rectangular QAM Demodulator Baseband/1 -> Rectangular QAM Modulator Baseband1/1, Unipolar to Bipolar Converter2/1
  General Block Deinterleaver1/1 -> Matrix Deinterleaver1/1
  Matrix Deinterleaver1/1 -> mscale out/1
  mscale/1 -> Matrix Multiply/1
  Matrix Multiply/1 -> Transpose/1
  Bits Per Symbol/1 -> Matrix Multiply/2
  Reshape6/1 -> General Block Deinterleaver1/1
  Transpose/1 -> Reshape6/1

== system ieee80211n/Demodbank/Demod_ss1/Demodulator 3 ==
  rxsig : Inport  Port=1  LatchInput=off
  mscale : Inport  Port=2  LatchInput=off
  Enable : EnablePort
  Bits Per Symbol : Constant  Value=ones(1, log2(modOrder))  VectorParams1D=off
  General Block Deinterleaver : commblkintrlv2/General Block Deinterleaver  elements=interleaverElements
  General Block Deinterleaver1 : commblkintrlv2/General Block Deinterleaver  elements=interleaverElements
  Matrix Deinterleaver : commblkintrlv2/Matrix Deinterleaver  Nrows=interleaverRows  Ncols=interleaverCols
  Matrix Deinterleaver1 : commblkintrlv2/Matrix Deinterleaver  Nrows=interleaverRows  Ncols=interleaverCols
  Matrix Multiply : Product  Multiplication=Matrix(*)
  Rectangular QAM Demodulator Baseband : commdigbbndam2/Rectangular QAM Demodulator Baseband  M=modOrder  OutType=Bit  Dec=Gray  PowType=Average Power  MinDist=2  AvgPow=1  PeakPow=1  Ph=0  numSamp=1
  Rectangular QAM Modulator Baseband1 : commdigbbndam2/Rectangular QAM Modulator Baseband  M=modOrder  InType=Bit  Enc=Gray  PowType=Average Power  MinDist=2  AvgPow=1  PeakPow=1  Ph=0  numSamp=1
  Reshape6 : simulink/Math Operations/Reshape  OutputDimensionality=Column vector  OutputDimensions=1600
  Sum : Sum  Inputs=|+-  SaturateOnIntegerOverflow=on
  Transpose : dspmtrx3/Transpose  Hermitian=off  overflowFlag=on
  Unipolar to Bipolar Converter2 : commutil2/Unipolar to Bipolar Converter  M=2  polarity=Negative
  rxdata : Outport  OutputWhenDisabled=reset  InitialOutput=0
  symerr : Outport  Port=2  OutputWhenDisabled=reset  InitialOutput=0
  mscale out : Outport  Port=3  OutputWhenDisabled=reset  InitialOutput=0
  wires:
  General Block Deinterleaver/1 -> Matrix Deinterleaver/1
  Matrix Deinterleaver/1 -> rxdata/1
  Sum/1 -> symerr/1
  Rectangular QAM Modulator Baseband1/1 -> Sum/1
  Unipolar to Bipolar Converter2/1 -> General Block Deinterleaver/1
  rxsig/1 -> Sum/2, Rectangular QAM Demodulator Baseband/1
  Rectangular QAM Demodulator Baseband/1 -> Rectangular QAM Modulator Baseband1/1, Unipolar to Bipolar Converter2/1
  General Block Deinterleaver1/1 -> Matrix Deinterleaver1/1
  Matrix Deinterleaver1/1 -> mscale out/1
  mscale/1 -> Matrix Multiply/1
  Matrix Multiply/1 -> Transpose/1
  Bits Per Symbol/1 -> Matrix Multiply/2
  Reshape6/1 -> General Block Deinterleaver1/1
  Transpose/1 -> Reshape6/1

== system ieee80211n/Demodbank/Demod_ss1/Demodulator 4 ==
  rxsig : Inport  Port=1  LatchInput=off
  mscale : Inport  Port=2  LatchInput=off
  Enable : EnablePort
  Bits Per Symbol : Constant  Value=ones(1, log2(modOrder))  VectorParams1D=off
  General Block Deinterleaver : commblkintrlv2/General Block Deinterleaver  elements=interleaverElements
  General Block Deinterleaver1 : commblkintrlv2/General Block Deinterleaver  elements=interleaverElements
  Matrix Deinterleaver : commblkintrlv2/Matrix Deinterleaver  Nrows=interleaverRows  Ncols=interleaverCols
  Matrix Deinterleaver1 : commblkintrlv2/Matrix Deinterleaver  Nrows=interleaverRows  Ncols=interleaverCols
  Matrix Multiply : Product  Multiplication=Matrix(*)
  Rectangular QAM Demodulator Baseband : commdigbbndam2/Rectangular QAM Demodulator Baseband  M=modOrder  OutType=Bit  Dec=Gray  PowType=Average Power  MinDist=2  AvgPow=1  PeakPow=1  Ph=0  numSamp=1
  Rectangular QAM Modulator Baseband1 : commdigbbndam2/Rectangular QAM Modulator Baseband  M=modOrder  InType=Bit  Enc=Gray  PowType=Average Power  MinDist=2  AvgPow=1  PeakPow=1  Ph=0  numSamp=1
  Reshape6 : simulink/Math Operations/Reshape  OutputDimensionality=Column vector  OutputDimensions=1600
  Sum : Sum  Inputs=|+-  SaturateOnIntegerOverflow=on
  Transpose : dspmtrx3/Transpose  Hermitian=off  overflowFlag=on
  Unipolar to Bipolar Converter2 : commutil2/Unipolar to Bipolar Converter  M=2  polarity=Negative
  rxdata : Outport  OutputWhenDisabled=reset  InitialOutput=0
  symerr : Outport  Port=2  OutputWhenDisabled=reset  InitialOutput=0
  mscale out : Outport  Port=3  OutputWhenDisabled=reset  InitialOutput=0
  wires:
  General Block Deinterleaver/1 -> Matrix Deinterleaver/1
  Matrix Deinterleaver/1 -> rxdata/1
  Sum/1 -> symerr/1
  Rectangular QAM Modulator Baseband1/1 -> Sum/1
  Unipolar to Bipolar Converter2/1 -> General Block Deinterleaver/1
  rxsig/1 -> Sum/2, Rectangular QAM Demodulator Baseband/1
  Rectangular QAM Demodulator Baseband/1 -> Rectangular QAM Modulator Baseband1/1, Unipolar to Bipolar Converter2/1
  General Block Deinterleaver1/1 -> Matrix Deinterleaver1/1
  Matrix Deinterleaver1/1 -> mscale out/1
  mscale/1 -> Matrix Multiply/1
  Matrix Multiply/1 -> Transpose/1
  Bits Per Symbol/1 -> Matrix Multiply/2
  Reshape6/1 -> General Block Deinterleaver1/1
  Transpose/1 -> Reshape6/1
